simulink model "iio_sink_sim"  (R2013b)
settings: Solver=ode45  StartTime=0.0  StopTime=inf  RelTol=1e-3
settings Model: Creator=ACozma  LastModifiedBy=ACozma

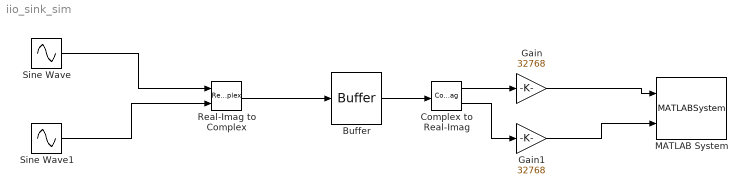
== system iio_sink_sim ==
  Buffer : Buffer  N=32768  TreatMby1Signals=One channel
  Complex to Real-Imag : ComplexToRealImag
  Gain : Gain  Gain=32768
  Gain1 : Gain  Gain=32768
  MATLAB System : MATLABSystem  System=iio_sink  SimulateUsing=Interpreted execution  src_ip_address=10.50.1.104  src_dev_name=cf-ad9361-dds-core-lpc  ch_size=32768  ch_no=2
      mask Type: iio_sink
      mask Display: disp('iio_sink');
  Real-Imag to Complex : RealImagToComplex
  Sine Wave : Sin  SineType=Sample based  Frequency=10  Samples=100  SampleTime=1
  Sine Wave1 : Sin  SineType=Sample based  Frequency=10  Phase=90  Samples=100  SampleTime=1  Offset=75
  wires:
  Complex to Real-Imag/1 -> Gain/1
  Complex to Real-Imag/2 -> Gain1/1
  Gain/1 -> MATLAB System/1
  Buffer/1 -> Complex to Real-Imag/1
  Sine Wave/1 -> Real-Imag to Complex/1
  Sine Wave1/1 -> Real-Imag to Complex/2
  Real-Imag to Complex/1 -> Buffer/1
  Gain1/1 -> MATLAB System/2
